simulink model "kinSwCtrl2"  (R2015a)
settings: Solver=ode45  StartTime=0.0  StopTime=sim_t  RelTol=1e-3
InitFcn:
  | set_kinSwCtrl2;
StopFcn:
  | plot_kinSwCtrl2;
values from neighbouring files (symbols this model uses):
  dlegAlp0 = -20*pi/180    (= -0.349065850399)    [set_kinSwCtrl2.m]
  kinSw_alpha_tgt = 70*pi/180    (= 1.2217304764)    [set_kinSwCtrl.m]    (also in set_kinSwCtrl2.m)
  kinSw_len_tgt = 0.8    [set_kinSwCtrl.m]    (also in set_kinSwCtrl2.m)
  kinSw_min_f_duration = kinSw_time_del*0.85    (= 0.425)    [set_kinSwCtrl.m]    (also in set_kinSwCtrl2.m)
  kinSw_time_del = 0.5    [set_kinSwCtrl.m]    (also in set_kinSwCtrl2.m)
  legAlp0 = 110*pi/180    (= 1.91986217719)    [set_kinSwCtrl2.m]
  legLen0 = 0.8    [set_kinSwCtrl2.m]
  test_t_SwStart = 0.001    [set_kinSwCtrl.m]    (also in set_kinSwCtrl2.m)
undefined symbols (not defined in the file or in its folder): kinSw_len_min
libraries: simulink x1
settings Model: Creator=smsong  LastModifiedBy=smsong

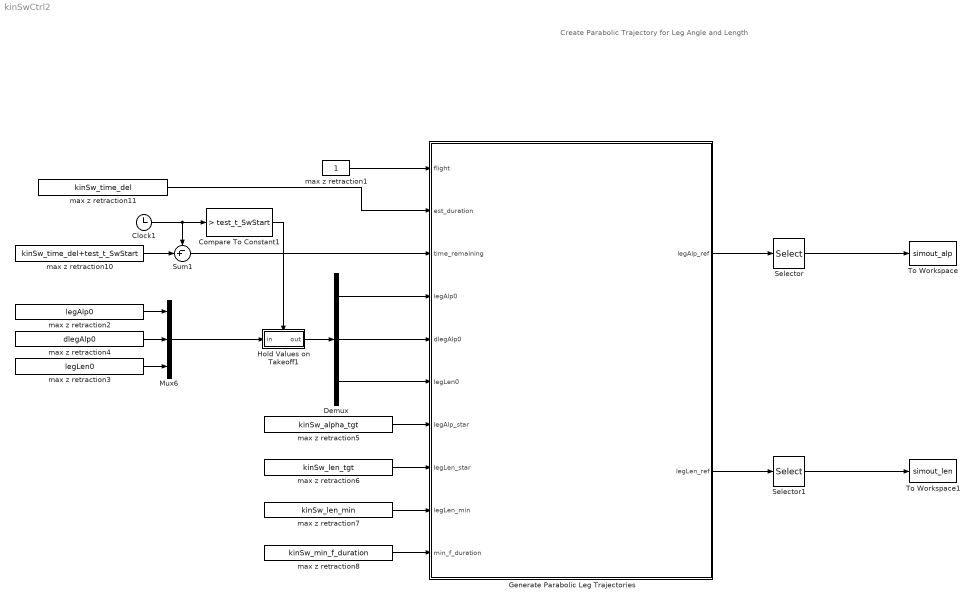
== system kinSwCtrl2 ==
  note: Create Parabolic
      | Trajectory for Leg Angle and Length
  Clock1 : Clock
  Compare To Constant1 : simulink/Logic and Bit Operations/Compare To Constant  relop=>  const=test_t_SwStart  OutDataTypeStr=boolean  ZeroCross=off
  Demux : Demux  Outputs=3
  Generate Parabolic Leg Trajectories : MATLAB Function  TreatAsAtomicUnit=on
  Hold Values on Takeoff1 : Subsystem
  Mux6 : Mux  Inputs=3
  Selector : Selector  InputPortWidth=3
  Selector1 : Selector  InputPortWidth=3
  Sum1 : Sum  Inputs=-+|
  To Workspace : ToWorkspace  VariableName=simout_alp  SaveFormat=Structure With Time  SampleTime=-1
  To Workspace1 : ToWorkspace  VariableName=simout_len  SaveFormat=Structure With Time  SampleTime=-1
  max z retraction1 : Constant
  max z retraction10 : Constant  Value=kinSw_time_del+test_t_SwStart
  max z retraction11 : Constant  Value=kinSw_time_del
  max z retraction2 : Constant  Value=legAlp0
  max z retraction3 : Constant  Value=legLen0
  max z retraction4 : Constant  Value=dlegAlp0
  max z retraction5 : Constant  Value=kinSw_alpha_tgt
  max z retraction6 : Constant  Value=kinSw_len_tgt
  max z retraction7 : Constant  Value=kinSw_len_min
  max z retraction8 : Constant  Value=kinSw_min_f_duration
  wires:
  Generate Parabolic Leg Trajectories/1(legAlp_ref) -> Selector/1
  Selector/1 -> To Workspace/1
  Selector1/1 -> To Workspace1/1
  max z retraction10/1 -> Sum1/2
  Clock1/1 -> Compare To Constant1/1, Sum1/1
  Sum1/1 -> Generate Parabolic Leg Trajectories/3(time_remaining)
  max z retraction1/1 -> Generate Parabolic Leg Trajectories/1(flight)
  max z retraction11/1 -> Generate Parabolic Leg Trajectories/2(est_duration)
  Generate Parabolic Leg Trajectories/2(legLen_ref) -> Selector1/1
  Compare To Constant1/1 -> Hold Values on Takeoff1/Trigger
  max z retraction2/1 -> Mux6/1
  Mux6/1 -> Hold Values on Takeoff1/1(in)
  Hold Values on Takeoff1/1(out) -> Demux/1
  Demux/1 -> Generate Parabolic Leg Trajectories/4(legAlp0)
  max z retraction3/1 -> Mux6/3
  max z retraction4/1 -> Mux6/2
  Demux/2 -> Generate Parabolic Leg Trajectories/5(dlegAlp0)
  Demux/3 -> Generate Parabolic Leg Trajectories/6(legLen0)
  max z retraction5/1 -> Generate Parabolic Leg Trajectories/7(legAlp_star)
  max z retraction6/1 -> Generate Parabolic Leg Trajectories/8(legLen_star)
  max z retraction7/1 -> Generate Parabolic Leg Trajectories/9(legLen_min)
  max z retraction8/1 -> Generate Parabolic Leg Trajectories/10(min_f_duration)

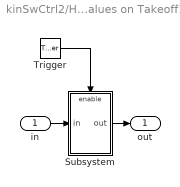
== system kinSwCtrl2/Hold Values on Takeoff1 ==
  in : Inport
  Trigger : TriggerPort  ShowOutputPort=on  PortDimensions=1
  Subsystem : Subsystem
  out : Outport
  wires:
  Trigger/1 -> Subsystem/Enable
  Subsystem/1(out) -> out/1
  in/1 -> Subsystem/1(in)

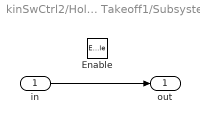
== system kinSwCtrl2/Hold Values on Takeoff1/Subsystem ==
  in : Inport
  Enable : EnablePort
  out : Outport
  wires:
  in/1 -> out/1

== matlab function kinSwCtrl2/Generate Parabolic Leg Trajectories ==
  data: flight input; est_duration input; time_remaining input; legAlp0 input; dlegAlp0 input; legLen0 input; legAlp_star input; legLen_star input; legLen_min input; legAlp_ref output size=3; legLen_ref output size=3; min_f_duration input
%% Parabolic trajectory generation for leg angle and length
% est_duration: estimated flight time
% time_remaining: time until estimated touchdown
% legAlp0: legAlp at takeoff
%   legAlp is the angle of attack
% legLen0: legLen at takeoff
% legAlp_star: desired legAlp
% legLen_star: desired legLen
% legLen_min: min legLen for ground clearance
% min_f_duration: minimum trajectory time

function [legAlp_ref, legLen_ref]  =  ...
          GenerateParabolicLegTrajectory(flight, ...
                    est_duration, time_remaining, ...
                    legAlp0, dlegAlp0, legLen0, legAlp_star, legLen_star, ...
                    legLen_min, min_f_duration)

if ~flight
    legAlp_ref = [0;0;0];
    legLen_ref = [0;0;0];
    return;
end

  % plan a traj from init to desired in estimated duration. Use a
  % discontinuous initial condition if estimated duration too short.
  duration = max(est_duration, min_f_duration);
  t_r = max(min(time_remaining, duration),0);   % !!!
  % sweep a parabola from x0 to x_star with dx_end = -dx0
  dlegAlp_star  = dlegAlp0;
  legAlp_star_t = legAlp_star + dlegAlp_star*t_r + (legAlp0-legAlp_star-dlegAlp_star*duration)*(t_r/duration)^2;
  dlegAlp_star_t = -dlegAlp_star - 2*(legAlp0-legAlp_star-dlegAlp_star*duration)*(t_r/duration^2);
  ddlegAlp_star_t =  2*(legAlp0-legAlp_star-dlegAlp_star*duration)*(1/duration^2);
  
  % Zero out velocities when out of time
  if time_remaining < 0
    dlegAlp_star_t = 0; ddlegAlp_star_t = 0;
  end 
  
  % split duration into thirds.  First segment: parabola from legLen0 to
  % legLen_min.  Second and third segments, cos to landing.
  dt3 = duration / 3;
  if t_r > 2*dt3;
    legLen_star_t = legLen_min + (legLen0-legLen_min)*((t_r-2*dt3)/dt3)^2;
    dlegLen_star_t = -(legLen0-legLen_min)*2*(t_r-2*dt3)/dt3/dt3;
    ddlegLen_star_t = (legLen0-legLen_min)*2/dt3^2;
  else
    legLen_star_t = legLen_star + (legLen_min-legLen_star)/2*(1-cos(t_r/(2*dt3)*pi));
    dlegLen_star_t = -(legLen_min-legLen_star)/2*sin(t_r/(2*dt3)*pi)*pi/(2*dt3);
    ddlegLen_star_t = (legLen_min-legLen_star)/2*cos(t_r/(2*dt3)*pi)*(pi/(2*dt3))^2;
  end
  
  % track a sinusoidal z of amplitude max_retract, finishing a half-cycle by t_end
  legAlp_ref = [legAlp_star_t; dlegAlp_star_t; ddlegAlp_star_t];
  legLen_ref = [legLen_star_t; dlegLen_star_t; ddlegLen_star_t];
